simulink model "ACC_Mode_Manager"  (R2024b)
settings: Solver=VariableStepAuto  StartTime=0.0  StopTime=10.0  RelTol=1e-3
settings Model: Creator=ezers  LastModifiedBy=ezers

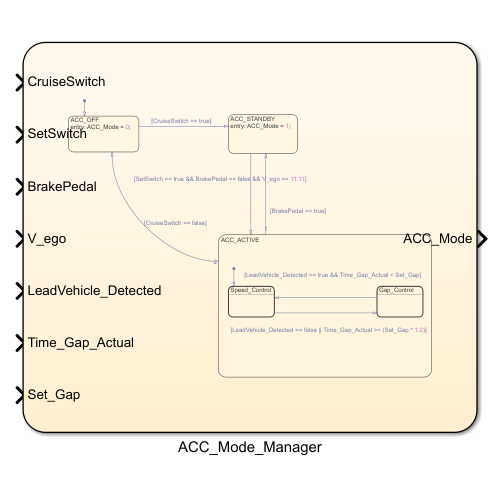
[thumbnail: Simulink's stored preview of the top-level diagram]
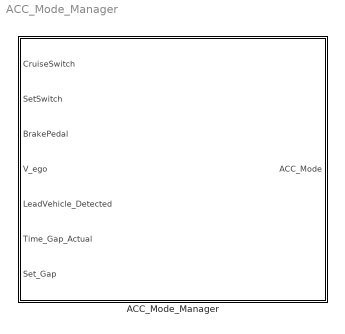
== system ACC_Mode_Manager ==
  ACC_Mode_Manager : Stateflow chart  TreatAsAtomicUnit=on

== stateflow chart ACC_Mode_Manager/ACC_Mode_Manager ==
  state ACC_STANDBY
    entry: ACC_Mode = 1;
  state ACC_OFF
    entry: ACC_Mode = 0;
  state ACC_ACTIVE
    state Speed_Control
      entry: ACC_Mode = 2;
    state Gap_Control
      entry: ACC_Mode = 3;
    (default) -> Speed_Control
    Gap_Control -> Speed_Control : [LeadVehicle_Detected == true && Time_Gap_Actual < Set_Gap]
    Speed_Control -> Gap_Control : [LeadVehicle_Detected == false || Time_Gap_Actual >= (Set_Gap * 1.2)]
  (default) -> ACC_OFF
  ACC_OFF -> ACC_STANDBY : [CruiseSwitch == true]
  ACC_ACTIVE -> ACC_OFF [order 2] : [CruiseSwitch == false]
  ACC_STANDBY -> ACC_ACTIVE : [SetSwitch == true && BrakePedal == false && V_ego >= 11.11]
  ACC_ACTIVE -> ACC_STANDBY [order 1] : [BrakePedal == true]
  data: CruiseSwitch input boolean; SetSwitch input boolean; BrakePedal input boolean; V_ego input double; LeadVehicle_Detected input boolean; Time_Gap_Actual input double; Set_Gap input double; ACC_Mode output uint8
  data CruiseSwitch settings: description=Bouton Master ON/OFF
  data SetSwitch settings: description=Bouton d'activation de la consigne
  data BrakePedal settings: description=État pédale de frein
  data V_ego settings: description=Vitesse véhicule hôte
  data LeadVehicle_Detected settings: description=Signal de présence (IA Perception)
  data Time_Gap_Actual settings: description=Temps inter-véhiculaire mesuré
  data Set_Gap settings: description=Consigne de sécurité (temps)
